simulink model "real_simulation"  (R2019b)
settings: Solver=VariableStepAuto  StartTime=0.0  StopTime=120.0  RelTol=1e-3
libraries: simulink x1
settings Model: Creator=logan  LastModifiedBy=logan
settings OptimizationCC: UseDivisionForNetSlopeComputation=on

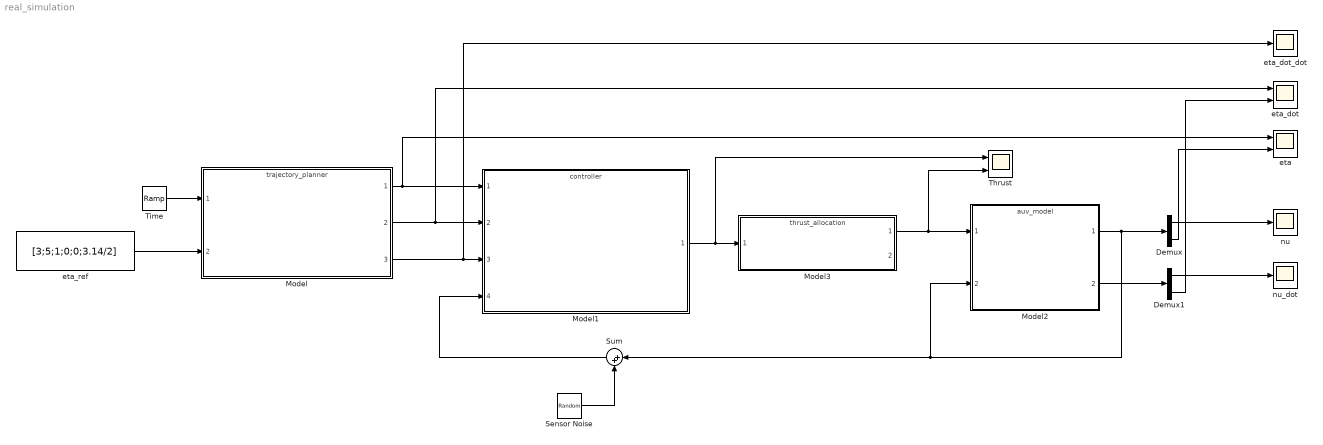
== system real_simulation ==
  Demux : Demux  Outputs=[6,6]
  Demux1 : Demux  Outputs=[6,6]
  Model : ModelReference  ModelNameDialog=trajectory_planner.slx  SimulationMode=Normal  ModelReferenceVersion=1.14
  Model1 : ModelReference  ModelNameDialog=controller.slx  SimulationMode=Normal  ModelReferenceVersion=1.52
  Model2 : ModelReference  ModelNameDialog=auv_model  SimulationMode=Normal  ModelReferenceVersion=1.6
  Model3 : ModelReference  ModelNameDialog=thrust_allocation.slx  SimulationMode=Normal  ModelReferenceVersion=1.30
  Sensor Noise : RandomNumber  Variance=0  SampleTime=1
  Sum : Sum  Inputs=|++
  Thrust : Scope  NumInputPorts=2
  "Time " : simulink/Sources/Ramp  slope=1  start=0  InitialOutput=0
  eta : Scope  NumInputPorts=2
  eta_dot : Scope  NumInputPorts=2
  eta_dot_dot : Scope
  eta_ref : Constant  Value=[3;5;1;0;0;3.14/2]
  nu : Scope
  nu_dot : Scope
  wires:
  Sum/1 -> Model1/4
  Demux/1 -> nu/1
  "Time "/1 -> Model/1
  Model2/2 -> Demux1/1
  Model/1 -> Model1/1, eta/1
  Demux1/2 -> eta_dot/2
  Model/2 -> eta_dot/1, Model1/2
  Model/3 -> eta_dot_dot/1, Model1/3
  eta_ref/1 -> Model/2
  Demux1/1 -> nu_dot/1
  Model2/1 -> Demux/1, Model2/2, Sum/1
  Sensor Noise/1 -> Sum/2
  Demux/2 -> eta/2
  Model1/1 -> Model3/1, Thrust/1
  Model3/1 -> Thrust/2, Model2/1
